simulink model "water_tank_p"  (R2024b)
settings: Solver=ode4  StartTime=0.0  StopTime=50  FixedStep=0.001  RelTol=1e-3
libraries: SignalEditorBlockLib x2
settings Model: Creator=max  LastModifiedBy=max

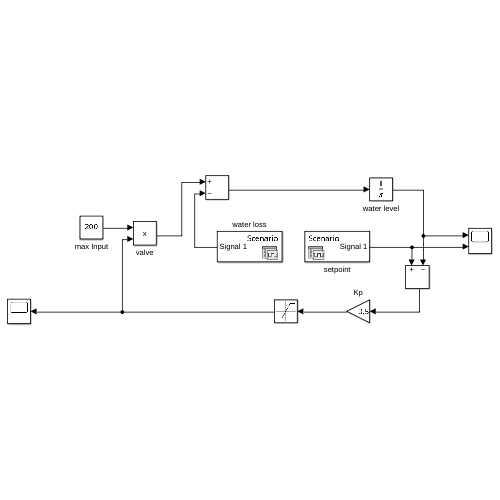
[thumbnail: Simulink's stored preview of the top-level diagram]
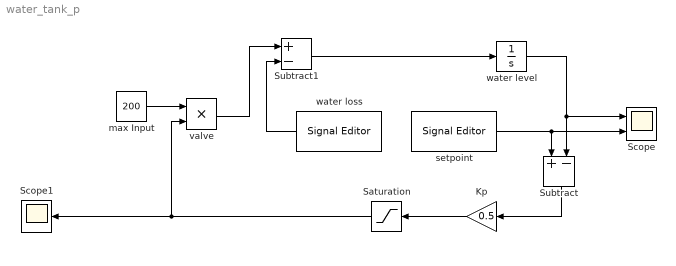
== system water_tank_p ==
  Kp : Gain  Gain=0.5
  Saturation : Saturate  UpperLimit=1  LowerLimit=0
  Scope : Scope  NumInputPorts=2
  Scope1 : Scope
  Subtract : Sum  Inputs=+-
  Subtract1 : Sum  Inputs=+-
  max Input : Constant  Value=200
  setpoint : SignalEditorBlockLib/Signal Editor  FileName=water_setpoint.mat  ActiveScenario=Scenario  ActiveSignal=Signal 1  IsBus=off  OutputBusObjectStr=Bus: BusObject  SampleTime=0  Interpolate=off  ZeroCross=off  OutputAfterFinalValue=Setting to zero  Unit=inherit  PreserveSignalName=on  ApplySigPropsToAllScenarios=on  ApplySigPropsToAllSignals=off
  valve : Product
  water level : Integrator  InitialCondition=1000
  water loss : SignalEditorBlockLib/Signal Editor  FileName=water_loss.mat  ActiveScenario=Scenario  ActiveSignal=Signal 1  IsBus=off  OutputBusObjectStr=Bus: BusObject  SampleTime=0  Interpolate=off  ZeroCross=off  OutputAfterFinalValue=Setting to zero  Unit=inherit  PreserveSignalName=on  ApplySigPropsToAllScenarios=on  ApplySigPropsToAllSignals=off
  wires:
  water level/1 -> Scope/1, Subtract/2
  setpoint/1 -> Scope/2, Subtract/1
  Subtract/1 -> Kp/1
  Kp/1 -> Saturation/1
  max Input/1 -> valve/1
  Saturation/1 -> Scope1/1, valve/2
  valve/1 -> Subtract1/1
  water loss/1 -> Subtract1/2
  Subtract1/1 -> water level/1
